simulink model "plant"  (R2021b)
settings: Solver=VariableStepAuto  StartTime=0.0  StopTime=10.0  RelTol=1e-3
undefined symbols (not defined in the file): k1, k2, m1, m2
libraries: simulink x1
settings Model: Creator=david  LastModifiedBy=david

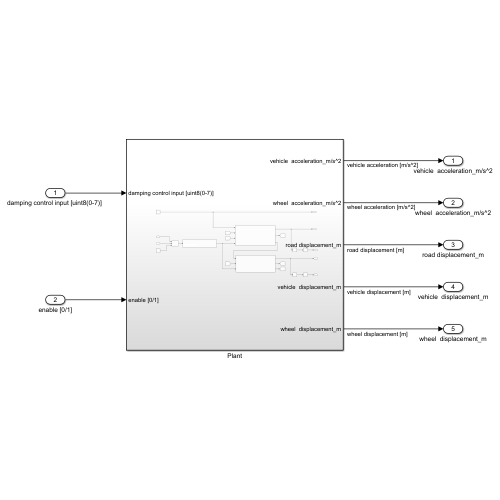
[thumbnail: Simulink's stored preview of the top-level diagram]
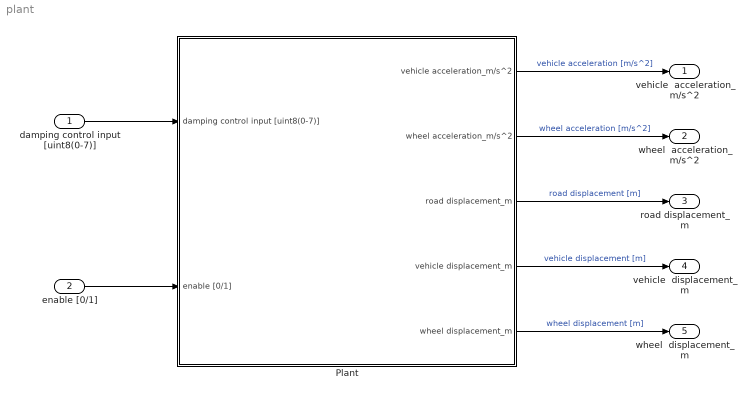
== system plant ==
  "damping control input [uint8(0-7)] " : Inport
  enable [0/1] : Inport  Port=2
  Plant : Subsystem
  vehicle  acceleration_m/s^2 : Outport  VectorParamsAs1DForOutWhenUnconnected=on
  wheel  acceleration_m/s^2 : Outport  Port=2  VectorParamsAs1DForOutWhenUnconnected=on
  road displacement_m : Outport  Port=3  VectorParamsAs1DForOutWhenUnconnected=on
  vehicle  displacement_m : Outport  Port=4  VectorParamsAs1DForOutWhenUnconnected=on
  wheel  displacement_m : Outport  Port=5  VectorParamsAs1DForOutWhenUnconnected=on
  wires:
  "damping control input [uint8(0-7)] "/1 -> Plant/1("damping control input [uint8(0-7)] ")
  enable [0/1]/1 -> Plant/2(enable [0/1])
  Plant/1(vehicle acceleration_m/s^2) -> vehicle  acceleration_m/s^2/1  "vehicle acceleration [m/s^2]"
  Plant/2(wheel acceleration_m/s^2) -> wheel  acceleration_m/s^2/1  "wheel acceleration [m/s^2]"
  Plant/3(road displacement_m) -> road displacement_m/1  "road displacement [m]"
  Plant/4(vehicle displacement_m) -> vehicle  displacement_m/1  "vehicle displacement [m]"
  Plant/5(wheel displacement_m) -> wheel  displacement_m/1  "wheel displacement [m]"

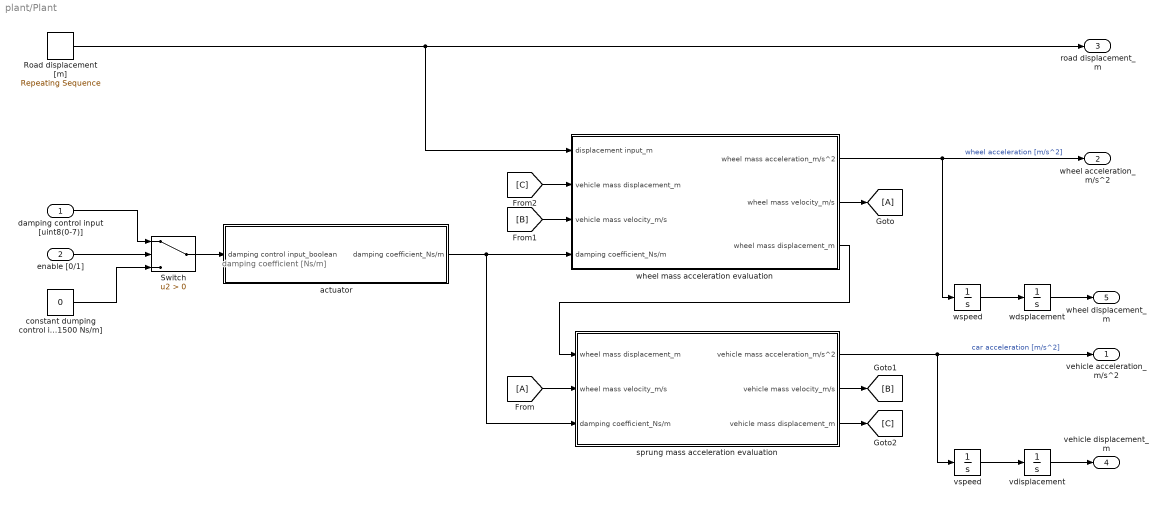
== system plant/Plant ==
  note: damping coefficient [Ns/m]
  "damping control input [uint8(0-7)] " : Inport  OutDataTypeStr=uint8
  enable [0/1] : Inport  Port=2
  Road displacement [m] : simulink/Sources/Repeating Sequence  rep_seq_t=[0 0.1 4 4.1 8 10 10.1 10.2 10.3 14]  rep_seq_y=[0 0.2 -0.2 0 -0.2 0 0.2 0.2 0 0]
  Switch : Switch  Criteria=u2 > Threshold
  actuator : Subsystem
  constant dumping control input [0=1500 Ns/m] : Constant  Value=0
  sprung mass acceleration evaluation : Subsystem
  vdisplacement : Integrator
  vspeed : Integrator
  wdsplacement : Integrator
  wheel mass acceleration evaluation : Subsystem
  wspeed : Integrator
  vehicle acceleration_m/s^2 : Outport
  wheel acceleration_m/s^2 : Outport  Port=2  Unit=m/s^2
  road displacement_m : Outport  Port=3  Unit=m
  vehicle displacement_m : Outport  Port=4  Unit=m
  wheel displacement_m : Outport  Port=5  Unit=m
  wires:
  Switch/1 -> actuator/1("damping control input_boolean ")
  actuator/1(damping coefficient_Ns/m) -> sprung mass acceleration evaluation/3(damping coefficient_Ns/m), wheel mass acceleration evaluation/4(damping coefficient_Ns/m)
  wheel mass acceleration evaluation/1(wheel mass acceleration_m/s^2) -> wheel acceleration_m/s^2/1, wspeed/1  "wheel acceleration [m/s^2]"
  wheel mass acceleration evaluation/2(wheel mass velocity_m/s) -> [A]
  sprung mass acceleration evaluation/1(vehicle mass acceleration_m/s^2) -> vehicle acceleration_m/s^2/1, vspeed/1  "car acceleration [m/s^2]"
  sprung mass acceleration evaluation/2(vehicle mass velocity_m/s) -> [B]
  enable [0/1]/1 -> Switch/2
  wspeed/1 -> wdsplacement/1
  [A] -> sprung mass acceleration evaluation/2(wheel mass velocity_m/s)
  vspeed/1 -> vdisplacement/1
  wdsplacement/1 -> wheel displacement_m/1
  constant dumping control input [0=1500 Ns/m]/1 -> Switch/3
  Road displacement [m]/1 -> road displacement_m/1, wheel mass acceleration evaluation/1(displacement input_m)
  wheel mass acceleration evaluation/3(wheel mass displacement_m) -> sprung mass acceleration evaluation/1(wheel mass displacement_m)
  "damping control input [uint8(0-7)] "/1 -> Switch/1
  vdisplacement/1 -> vehicle displacement_m/1
  [B] -> wheel mass acceleration evaluation/3(vehicle mass velocity_m/s)
  sprung mass acceleration evaluation/3(vehicle mass displacement_m) -> [C]
  [C] -> wheel mass acceleration evaluation/2(vehicle mass displacement_m)

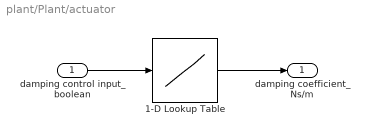
== system plant/Plant/actuator ==
  "damping control input_boolean " : Inport
  1-D Lookup Table : Lookup_n-D  NumberOfTableDimensions=1  BreakpointsForDimension1=uint8([0,1]);  Table=[1500,6000]  InternalRulePriority=Speed  RndMeth=Simplest  InputSameDT=on
  damping coefficient_Ns/m : Outport  Unit=N*second/m
  wires:
  "damping control input_boolean "/1 -> 1-D Lookup Table/1
  1-D Lookup Table/1 -> damping coefficient_Ns/m/1

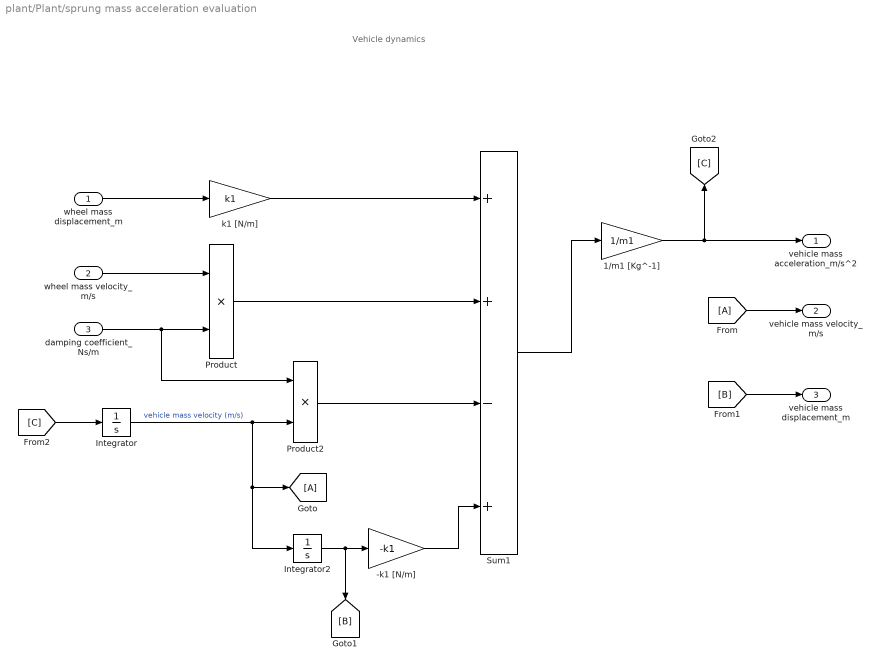
== system plant/Plant/sprung mass acceleration evaluation ==
  note: Vehicle dynamics
  wheel mass displacement_m : Inport
  wheel mass velocity_m/s : Inport  Port=2
  damping coefficient_Ns/m : Inport  Port=3  Unit=N*s/m
  -k1 [N/m] : Gain  Gain=-k1
  1/m1 [Kg^-1] : Gain  Gain=1/m1
  Integrator : Integrator
  Integrator2 : Integrator
  Product : Product
  Product2 : Product
  Sum1 : Sum  Inputs=++-+
  k1 [N/m] : Gain  Gain=k1
  vehicle mass acceleration_m/s^2 : Outport  Unit=m/s^2
  vehicle mass velocity_m/s : Outport  Port=2  Unit=m/s
  vehicle mass displacement_m : Outport  Port=3  Unit=m
  wires:
  Sum1/1 -> 1/m1 [Kg^-1]/1
  Integrator/1 -> Integrator2/1, [A], Product2/2  "vehicle mass velocity (m/s)"
  Integrator2/1 -> [B], -k1 [N/m]/1
  wheel mass displacement_m/1 -> k1 [N/m]/1
  wheel mass velocity_m/s/1 -> Product/1
  damping coefficient_Ns/m/1 -> Product2/1, Product/2
  k1 [N/m]/1 -> Sum1/1
  Product/1 -> Sum1/2
  Product2/1 -> Sum1/3
  1/m1 [Kg^-1]/1 -> [C], vehicle mass acceleration_m/s^2/1
  -k1 [N/m]/1 -> Sum1/4
  [A] -> vehicle mass velocity_m/s/1
  [B] -> vehicle mass displacement_m/1
  [C] -> Integrator/1

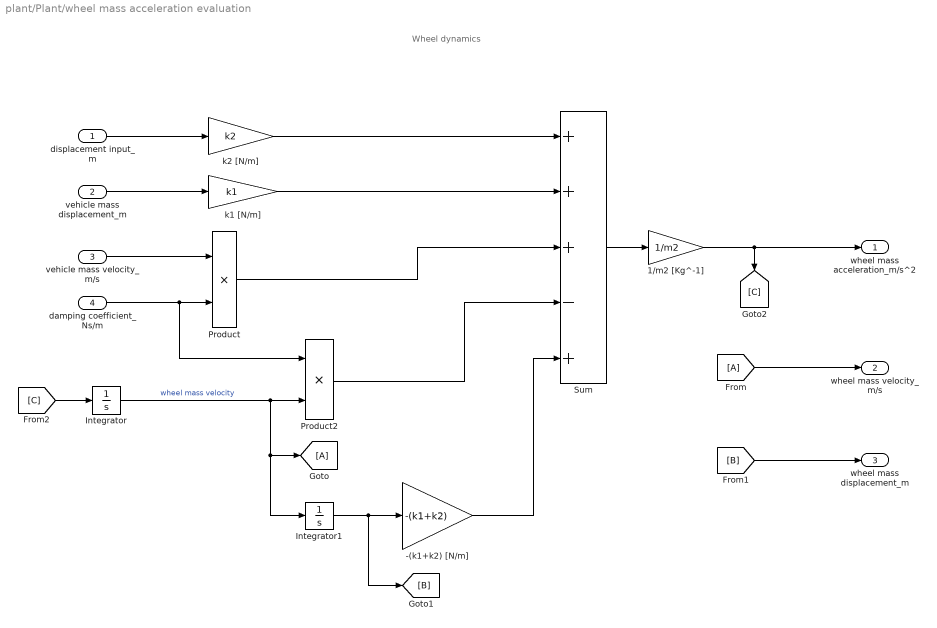
== system plant/Plant/wheel mass acceleration evaluation ==
  note: Wheel dynamics
  displacement input_m : Inport  OutDataTypeStr=double  Unit=m
  vehicle mass displacement_m : Inport  Port=2  Unit=m
  vehicle mass velocity_m/s : Inport  Port=3  Unit=m/s
  damping coefficient_Ns/m : Inport  Port=4  Unit=N*sec/m
  -(k1+k2) [N/m] : Gain  Gain=-(k1+k2)
  1/m2 [Kg^-1] : Gain  Gain=1/m2
  Integrator : Integrator
  Integrator1 : Integrator
  Product : Product
  Product2 : Product
  Sum : Sum  Inputs=+++-+
  k1 [N/m] : Gain  Gain=k1
  k2 [N/m] : Gain  Gain=k2
  wheel mass acceleration_m/s^2 : Outport  Unit=m/s^2
  wheel mass velocity_m/s : Outport  Port=2  Unit=m/s
  wheel mass displacement_m : Outport  Port=3  Unit=m
  wires:
  Sum/1 -> 1/m2 [Kg^-1]/1
  k2 [N/m]/1 -> Sum/1
  Integrator/1 -> [A], Integrator1/1, Product2/2  "wheel mass velocity"
  Integrator1/1 -> [B], -(k1+k2) [N/m]/1
  vehicle mass displacement_m/1 -> k1 [N/m]/1
  displacement input_m/1 -> k2 [N/m]/1
  vehicle mass velocity_m/s/1 -> Product/1
  damping coefficient_Ns/m/1 -> Product2/1, Product/2
  k1 [N/m]/1 -> Sum/2
  Product/1 -> Sum/3
  Product2/1 -> Sum/4
  -(k1+k2) [N/m]/1 -> Sum/5
  1/m2 [Kg^-1]/1 -> wheel mass acceleration_m/s^2/1, [C]
  [A] -> wheel mass velocity_m/s/1
  [B] -> wheel mass displacement_m/1
  [C] -> Integrator/1
